simulink model "test"  (R2015b)
settings: Solver=FixedStepDiscrete  StartTime=0.0  StopTime=inf  FixedStep=0.05  RelTol=1e-3
libraries: arduino_io_lib x3, arduinolib x1, simulink x1
settings Model: SimulationMode=external  ExtModeTrigDuration=2  Creator=yyas16  LastModifiedBy=yyas16
settings OptimizationCC: OptimizeModelRefInitCode=on  LifeSpan=Inf  MaxStackSize=64
settings HardwareCC: ProdBitPerInt=16  ProdBitPerPointer=16  ProdLargestAtomicFloat=None  ProdWordSize=8  ProdHWDeviceType=Atmel->AVR
settings RTWCC: SystemTargetFile=ert.tlc  TemplateMakefile=ert_default_tmf  Description=Embedded Coder  Toolchain=Arduino AVR v1.6.1  BuildConfiguration=Faster Runs
settings CodeAppCC: IgnoreCustomStorageClasses=off

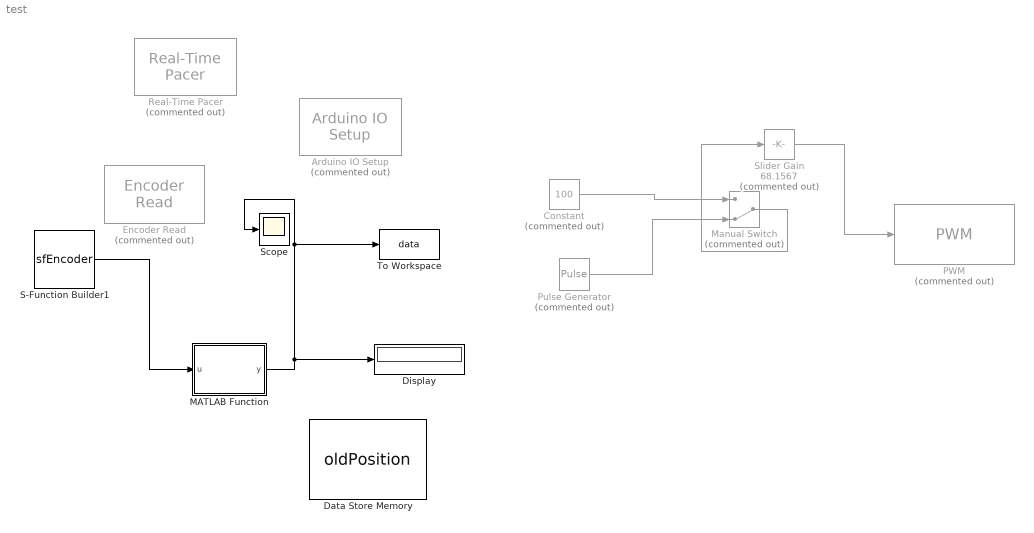
== system test ==
  Arduino IO Setup : arduino_io_lib/Arduino IO Setup  Priority=3  Commented=on  arduinoVar=Temporary arduino variable: Arduino1  workspaceVarName=a  comPort=/dev/cu.usbmodem1411
  Constant : Constant  Commented=on  Value=100
  Data Store Memory : DataStoreMemory  DataStoreName=oldPosition  ReadBeforeWriteMsg=warning  WriteAfterWriteMsg=warning  WriteAfterReadMsg=warning  OutDataTypeStr=int32
  Display : Display
  Encoder Read : arduino_io_lib/Encoder Read  Commented=on  arduinoVar=Temporary arduino variable: Arduino1  encNum=1  pinA=3  pinB=2  DbDl=0  T=0.2
  MATLAB Function : MATLAB Function  TreatAsAtomicUnit=on
  Manual Switch : ManualSwitch  Commented=on  CurrentSetting=0
  PWM : arduinolib/PWM  Commented=on  pinNumber=13  blockPlatform=arduino
  Pulse Generator : DiscretePulseGenerator  Commented=on  PulseType=Time based  Period=0.02  PulseWidth=50
  Real-Time Pacer : arduino_io_lib/Real-Time Pacer  Commented=on  simTimePerRealTime=20
  S-Function Builder1 : S-Function  InitFcn=try, set_param(gcb,'FunctionName','sfEncoder'), end  FunctionName=sfEncoder  Parameters=uint8(2),uint8(3)  SFunctionModules=sfEncoder_wrapper  SFunctionDeploymentMode=off  EnableBusSupport=off  mask(S-Function Builder){}
      mask help: Simulink:masks:SFunctionBuilder_MD
      mask init:
      | val = [[.9  0.75 0.75 1 1 .9 .9 1]',[1 1 0.75 0.75 .9 .9 1 .9]'];try , sys = get_param(gcb,'SfunBuilderFcnName');if isempty(sys), sys = get_param(gcb,'FunctionName'); end,catch, sys = get_param(gcb,'FunctionName'); end
      settings: CopyFcn=set_param(gcbh,'LinkStatus','none')  PreSaveFcn=try, set_param(gcb,'FunctionName','sfEncoder'), end  OpenFcn=sfunctionwizard(gcbh)
      mask Display: plot(val(:,1),val(:,2)),disp(sys), port_label('output',1,'counts')
  Scope : Scope
  Slider Gain : simulink/Math Operations/Slider Gain  Commented=on  low=0  gain=68.1567  high=255
  To Workspace : ToWorkspace  VariableName=data  SaveFormat=Timeseries  SampleTime=-1
  wires:
  Constant/1 -> Manual Switch/1
  Pulse Generator/1 -> Manual Switch/2
  Manual Switch/1 -> Slider Gain/1
  Slider Gain/1 -> PWM/1
  S-Function Builder1/1 -> MATLAB Function/1(u)
  MATLAB Function/1(y) -> To Workspace/1, Scope/1, Display/1

== matlab function test/MATLAB Function ==
  data: u input; y output double; oldPosition data_store_memory
function y = fcn(u)
%#codegen
global oldPosition

dt = 0.05; % sampling rate
ratio = 4 * 5 * 10; % gear ratioや４逓倍

temp = ( double(u) - double(oldPosition));
y = temp * 360.0 / ratio / dt;
% y  = u;
oldPosition = u;
